simulink model "control_rodilla_simulink"  (R2024a)
settings: Solver=VariableStepAuto  StartTime=0.0  StopTime=4  RelTol=1e-3
values from neighbouring files (symbols this model uses):
  b_pass = 0.05    [control_rodilla_mvp.m]    (also in parametros_control_rodilla.m)
  Bs = 1.0    (= 1)    [control_rodilla_mvp.m]    (also in parametros_control_rodilla.m)
  k_pass = 0.5    [control_rodilla_mvp.m]    (also in parametros_control_rodilla.m)
  Ks = 8    [control_rodilla_mvp.m]    (also in parametros_control_rodilla.m)
  L = casos(i,2)    [control_rodilla_mvp.m]    (also in parametros_control_rodilla.m = 0.42)
  M = casos(i,1)    [control_rodilla_mvp.m]    (also in parametros_control_rodilla.m = 25)
  torque_lim = 29.4    [control_rodilla_mvp.m]    (also in parametros_control_rodilla.m)
settings Model: Creator=MARIEL  LastModifiedBy=MARIEL

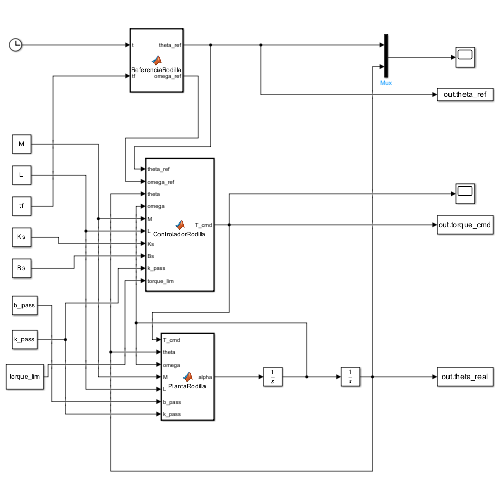
[thumbnail: Simulink's stored preview of the top-level diagram]
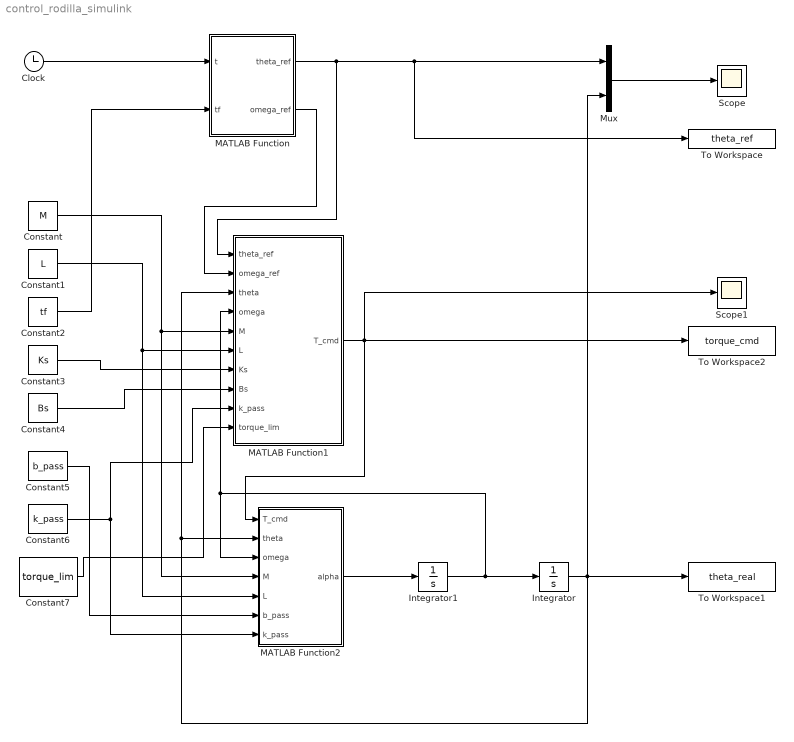
== system control_rodilla_simulink ==
  Clock : Clock
  Constant : Constant  Value=M
  Constant1 : Constant  Value=L
  Constant2 : Constant  Value=tf
  Constant3 : Constant  Value=Ks
  Constant4 : Constant  Value=Bs
  Constant5 : Constant  Value=b_pass
  Constant6 : Constant  Value=k_pass
  Constant7 : Constant  Value=torque_lim
  Integrator : Integrator
  Integrator1 : Integrator
  MATLAB Function : MATLAB Function  TreatAsAtomicUnit=on
  MATLAB Function1 : MATLAB Function  TreatAsAtomicUnit=on
  MATLAB Function2 : MATLAB Function  TreatAsAtomicUnit=on
  Mux : Mux  Inputs=2
  Scope : Scope
  Scope1 : Scope
  To Workspace : ToWorkspace  VariableName=theta_ref  SaveFormat=Timeseries  SampleTime=-1
  To Workspace1 : ToWorkspace  VariableName=theta_real  SaveFormat=Timeseries  SampleTime=-1
  To Workspace2 : ToWorkspace  VariableName=torque_cmd  SaveFormat=Timeseries  SampleTime=-1
  wires:
  MATLAB Function2/1(alpha) -> Integrator1/1
  Clock/1 -> MATLAB Function/1(t)
  Constant2/1 -> MATLAB Function/2(tf)
  MATLAB Function/1(theta_ref) -> MATLAB Function1/1(theta_ref), To Workspace/1, Mux/1
  MATLAB Function/2(omega_ref) -> MATLAB Function1/2(omega_ref)
  Constant/1 -> MATLAB Function2/4(M), MATLAB Function1/5(M)
  Constant1/1 -> MATLAB Function2/5(L), MATLAB Function1/6(L)
  Constant3/1 -> MATLAB Function1/7(Ks)
  Constant4/1 -> MATLAB Function1/8(Bs)
  Constant6/1 -> MATLAB Function1/9(k_pass), MATLAB Function2/7(k_pass)
  MATLAB Function1/1(T_cmd) -> Scope1/1, To Workspace2/1, MATLAB Function2/1(T_cmd)
  Integrator1/1 -> MATLAB Function1/4(omega), MATLAB Function2/3(omega), Integrator/1
  Integrator/1 -> To Workspace1/1, Mux/2, MATLAB Function2/2(theta), MATLAB Function1/3(theta)
  Constant5/1 -> MATLAB Function2/6(b_pass)
  Constant7/1 -> MATLAB Function1/10(torque_lim)
  Mux/1 -> Scope/1

== matlab function control_rodilla_simulink/MATLAB Function1 ==
  data: theta_ref input; T_cmd output; omega_ref input; theta input; omega input; M input; L input; Ks input; Bs input; k_pass input; torque_lim input
function T_cmd = ControladorRodilla(theta_ref, omega_ref, theta, omega, M, L, Ks, Bs, k_pass, torque_lim)

g = 9.81;
factor_CM = 0.43;
porcentaje_pierna_pie = 0.06;
theta0 = 0;

m = porcentaje_pierna_pie * M;
d = factor_CM * L;

% Compensación aproximada de gravedad y rigidez
T_grav_ref = m*g*d*sin(theta_ref);
T_rig_ref = k_pass*(theta_ref - theta0);

% Control de rigidez/impedancia simplificado
T_unsat = T_grav_ref + T_rig_ref + ...
          Ks*(theta_ref - theta) + ...
          Bs*(omega_ref - omega);

% Saturación del actuador
if T_unsat > torque_lim
    T_cmd = torque_lim;
elseif T_unsat < -torque_lim
    T_cmd = -torque_lim;
else
    T_cmd = T_unsat;
end

end

== matlab function control_rodilla_simulink/MATLAB Function ==
  data: t input; theta_ref output; tf input; omega_ref output
function [theta_ref, omega_ref] = ReferenciaRodilla(t, tf)

theta_i = deg2rad(0);
theta_f = deg2rad(90);

u = t/tf;

if u > 1
    u = 1;
end

if u < 0
    u = 0;
end

% Trayectoria suave minimum jerk
s = 10*u^3 - 15*u^4 + 6*u^5;
sdot = (30*u^2 - 60*u^3 + 30*u^4)/tf;

delta_theta = theta_f - theta_i;

theta_ref = theta_i + delta_theta*s;
omega_ref = delta_theta*sdot;

end

== matlab function control_rodilla_simulink/MATLAB Function2 ==
  data: T_cmd input; alpha output; theta input; omega input; M input; L input; b_pass input; k_pass input
function alpha = PlantaRodilla(T_cmd, theta, omega, M, L, b_pass, k_pass)

g = 9.81;
factor_CM = 0.43;
porcentaje_pierna_pie = 0.06;
theta0 = 0;

m = porcentaje_pierna_pie * M;
d = factor_CM * L;

% Inercia aproximada del segmento pierna-pie
I = m*d^2;

% Torques resistentes
T_grav = m*g*d*sin(theta);
T_fric = b_pass*omega;
T_rig = k_pass*(theta - theta0);

% Dinámica angular
alpha = (T_cmd - T_grav - T_fric - T_rig)/I;

end
